simulink model "full_state_linearized_model"  (R2024b)
settings: Solver=VariableStepAuto  StartTime=0.0  StopTime=100  FixedStep=1e-3  RelTol=1e-4
values from neighbouring files (symbols this model uses):
  A = [0 0 0 0 0 0 3.27333333333 13.0933333333 1 0 -0.00666666666667 -0.00666666666667 ... (16 elements, 4x4)]    [C_sisotool.mat]    (also in SystemAnalysis.m = [0     0               1                 0; matlab.mat)
  B = [0 0 0.666666666667 0.666666666667]    [C_sisotool.mat]    (also in SystemAnalysis.m = [0 0 1/mc 1/(L*mc)]'; matlab.mat)
undefined symbols (not defined in the file or in its folder): K
settings Model: Creator=pedro  LastModifiedBy=pedro

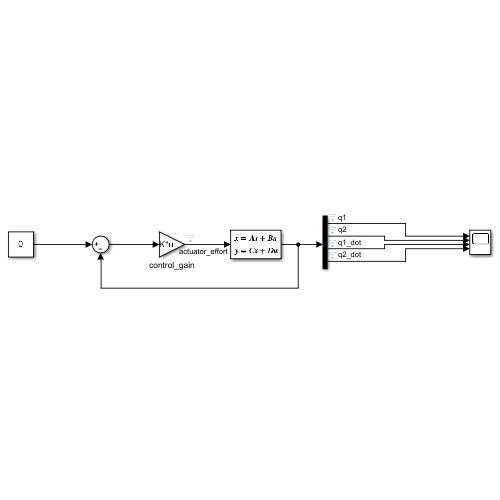
[thumbnail: Simulink's stored preview of the top-level diagram]
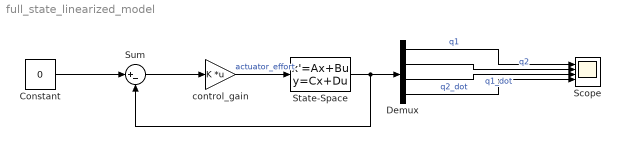
== system full_state_linearized_model ==
  Constant : Constant  Value=0
  Demux : Demux
  Scope : Scope  NumInputPorts=4
  State-Space : StateSpace  A=A  B=B  C=eye(4,4)  D=zeros(4,1)  InitialCondition=deg2rad(10)
  Sum : Sum  Inputs=|+-
  control_gain : Gain  Gain=K  Multiplication=Matrix(K*u)
  wires:
  State-Space/1 -> Sum/2, Demux/1
  Demux/1 -> Scope/1  "q1"
  Demux/2 -> Scope/2  "q2"
  Demux/3 -> Scope/3  "q1_dot"
  Demux/4 -> Scope/4  "q2_dot"
  Constant/1 -> Sum/1
  control_gain/1 -> State-Space/1  "actuator_effort"
  Sum/1 -> control_gain/1
